simulink model "New_heat_capacity"  (Simulink 7.9)
settings: Solver=FixedStepDiscrete  StartTime=0.0  StopTime=10  FixedStep=1  RelTol=1e-3
undefined symbols (not defined in the file): Carnot_heat_capacity_Callbacks
settings Model: Creator=awohlfei  LastModifiedBy=awohlfei

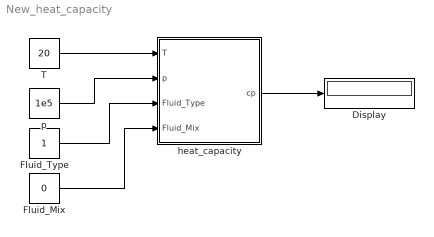
== system New_heat_capacity ==
  Display : Display
  Fluid_Mix : Constant  Value=0
  Fluid_Type : Constant
  T : Constant  Value=20
  heat_capacity : Subsystem  LoadFcn=Carnot_heat_capacity_Callbacks('LoadFcn');  InitFcn=load('THB.mat');  VariantObject=CarlibClassic  mask(heat capacity){INPUTARGUMENTS=state variables (classic), DEBUGLEVEL=WARNING, MAXTOTALWARNINGS=inf, MAXCONSECUTIVEWARNINGS=inf, WRITETOFILE=0, FILENAME='errors.txt'}
      mask prompts: INPUTARGUMENTS "Input arguments"; DEBUGLEVEL "Debug level"; MAXTOTALWARNINGS "maximum number of total warning"; MAXCONSECUTIVEWARNINGS "maximum number of consecutive warnings"; WRITETOFILE "write messages to file"; FILENAME "filename for error messages"
      mask help:
      | Calculates the  heat_capacity of fluids [J/(kg*K)].
      | Calls calls the function "heat_capacity" in the CARNOT library "carlib".
      mask init:
      | %Inports
      | Carnot_heat_capacity_Callbacks('CreateInports');
      | 
      | %global debug level
      | [DEBUGLEVEL, MAXTOTALWARNINGS, MAXCONSECUTIVEWARNINGS, WRITETOFILE, FILENAME] = Carnot_heat_capacity_Callbacks('CheckDebugLevels', DEBUGLEVEL, MAXTOTALWARNINGS, MAXCONSECUTIVEWARNINGS, WRITETOFILE, FILENAME);
      mask StyleString: popup(state variables (classic)|THB|THV),popup(DEBUG|INFO|WARNING|ERROR|FATAL|NONE),edit,edit,edit,edit
      mask CallbackString: Carnot_heat_capacity_Callbacks('MaskVisibilities');|||||
      mask TabNameString: Parameters,Debugging,Debugging,Debugging,Debugging,Debugging
  p : Constant  Value=1e5
  wires:
  T/1 -> heat_capacity/1(T)
  p/1 -> heat_capacity/2(p)
  Fluid_Type/1 -> heat_capacity/3(Fluid_Type)
  Fluid_Mix/1 -> heat_capacity/4(Fluid_Mix)
  heat_capacity/1(cp) -> Display/1

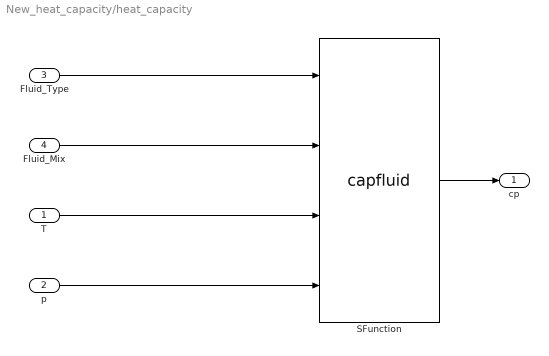
== system New_heat_capacity/heat_capacity ==
  T : Inport
  p : Inport  Port=2
  Fluid_Type : Inport  Port=3
  Fluid_Mix : Inport  Port=4
  SFunction : S-Function  FunctionName=capfluid  Parameters=DEBUGLEVEL,MAXTOTALWARNINGS,MAXCONSECUTIVEWARNINGS,WRITETOFILE,FILENAME  EnableBusSupport=off
  cp : Outport
  wires:
  SFunction/1 -> cp/1
  T/1 -> SFunction/3
  p/1 -> SFunction/4
  Fluid_Type/1 -> SFunction/1
  Fluid_Mix/1 -> SFunction/2
